simulink model "FA_18_MPC_Controller_2016b"  (R2016b)
settings: Solver=ode45  StartTime=0.0  StopTime=200  RelTol=1e-3
PreLoadFcn:
  | F18_Linear
values from neighbouring files (symbols this model uses):
  C1 = [0 -1 0 1]    [F18_Linear.m]
  d2r = pi/180    (= 0.0174532925199)    [F18_Linear.m]    (also in FA_18_Trim.m; FA_18_sfun.m; Sim.m)
  F1 = [-67.81 11973 -133.3 -11801]    [F18_Linear.m]
  F2 = 1414.2    [F18_Linear.m]
  Trimx_N = [365.74;15*d2r;0;15*d2r]    [F18_Linear.m]
undefined symbols (not defined in the file or in its folder): Earth, WGS84
libraries: simulink_extras x2, aerolibfltsims x1, mpclib x1, aerolibtransform2 x1, aerolibconvert2 x1
settings Model: Creator=User  LastModifiedBy=Amruth Nanjangud

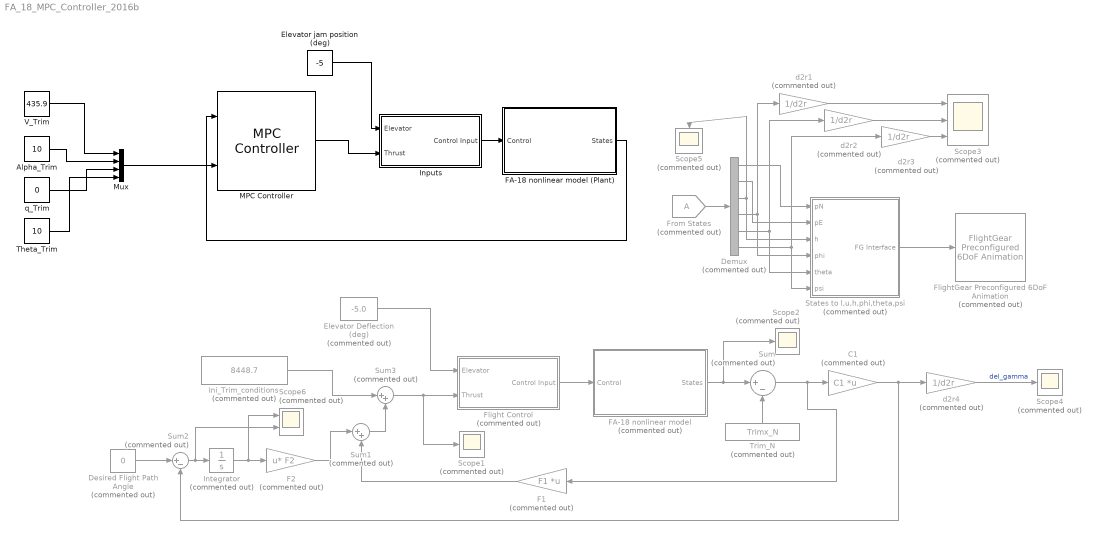
== system FA_18_MPC_Controller_2016b ==
  Alpha_Trim : Constant  Value=10
  C1 : Gain  Commented=on  Gain=C1  Multiplication=Matrix(K*u)
  Demux : Demux  Commented=on  Outputs=6
  Desired Flight Path Angle : Constant  Commented=on  Value=0
  Elevator Deflection (deg) : Constant  Commented=on  Value=-5.0
  Elevator jam position (deg) : Constant  Value=-5
  F1 : Gain  Commented=on  Gain=F1  Multiplication=Matrix(K*u)
  F2 : Gain  Commented=on  Gain=F2  Multiplication=Matrix(u*K)
  FA-18 nonlinear model : Subsystem  Commented=on
  FA-18 nonlinear model (Plant) : Subsystem
  Flight Control : Subsystem  Commented=on
  FlightGear Preconfigured 6DoF Animation : aerolibfltsims/FlightGear Preconfigured 6DoF Animation  Commented=on  xFlightGearVersion=v2016.1  DestinationIpAddress=127.0.0.1  DestinationPort=5502  SampleTime=1/30
  From States : From  Commented=on  TagVisibility=global
  Ini_Trim_conditions : Constant  Commented=on  Value=8448.7
  "Inputs " : Subsystem
  Integrator : Integrator  Commented=on
  MPC Controller : mpclib/MPC Controller  SCDEnableBlockLinearizationSpecification=on  mpcobj=mpc1  is_multiple=0  enable_value=0  return_u0=off  ref_from_ws=off  ref_signal_name=[]  ref_preview=off  md_from_ws=off  md_signal_name=[]  md_preview=off  from_project=off  project_file=MPCtask.mat  md_inport=off  mv_inport=off  cost_outport=off  return_sequence=off  return_qpstatus=off  return_state=off  state_inport=off  lims_inport=off  ywt_inport=off  is_designfromscratch=0  uwt_inport=off  duwt_inport=off  rhoeps_inport=off  uref_inport=off  n_ts=0.1  n_mv=1  n_md=0  n_ud=0  n_mo=4  n_uo=0  BlockDataType=double  SampleTimeInherited=off  switch_inport=off
  Mux : Mux
  Scope{1..2,4..5} (4 alike) : Scope  Commented=on
  Scope3 : Scope  Commented=on  NumInputPorts=3
  Scope6 : Scope  Commented=on  NumInputPorts=2
  States to l,u,h,phi,theta,psi : Subsystem  Commented=on
  Sum : Sum  Commented=on  Inputs=|+-
  Sum1 : Sum  Commented=on  Inputs=|++
  Sum2 : Sum  Commented=on  Inputs=|+-
  Sum3 : Sum  Commented=on  Inputs=|++
  Theta_Trim : Constant  Value=10
  Trim_N : Constant  Commented=on  Value=Trimx_N
  V_Trim : Constant  Value=435.9
  d2r{1..4} (4 alike) : Gain  Commented=on  Gain=1/d2r
  q_Trim : Constant  Value=0
  wires:
  Flight Control/1(Control Input) -> FA-18 nonlinear model/1(Control)
  Elevator Deflection (deg)/1 -> Flight Control/1(Elevator)
  FA-18 nonlinear model/1(States) -> Scope2/1, Sum/1
  Trim_N/1 -> Sum/2
  d2r4/1 -> Scope4/1  "del_gamma"
  Sum2/1 -> Scope6/2, Integrator/1
  Integrator/1 -> Scope6/1, F2/1
  Desired Flight Path Angle/1 -> Sum2/1
  C1/1 -> d2r4/1, Sum2/2
  F2/1 -> Sum1/1
  Sum1/1 -> Sum3/2
  F1/1 -> Sum1/2
  Sum3/1 -> Scope1/1, Flight Control/2(Thrust)
  Ini_Trim_conditions/1 -> Sum3/1
  Sum/1 -> F1/1, C1/1
  States to l,u,h,phi,theta,psi/1(FG Interface) -> FlightGear Preconfigured 6DoF Animation/1
  From States/1 -> Demux/1
  Demux/1 -> States to l,u,h,phi,theta,psi/1(pN)
  Demux/2 -> States to l,u,h,phi,theta,psi/2(pE)
  Demux/5 -> States to l,u,h,phi,theta,psi/5(theta), d2r2/1
  Demux/6 -> d2r3/1, States to l,u,h,phi,theta,psi/6(psi)
  Demux/4 -> d2r1/1, States to l,u,h,phi,theta,psi/4(phi)
  d2r1/1 -> Scope3/1
  d2r2/1 -> Scope3/2
  d2r3/1 -> Scope3/3
  Demux/3 -> Scope5/1, States to l,u,h,phi,theta,psi/3(h)
  "Inputs "/1(Control Input) -> FA-18 nonlinear model (Plant)/1(Control)
  MPC Controller/1 -> "Inputs "/2(Thrust)
  Elevator jam position (deg)/1 -> "Inputs "/1(Elevator)
  FA-18 nonlinear model (Plant)/1(States) -> MPC Controller/1
  Mux/1 -> MPC Controller/2
  V_Trim/1 -> Mux/1
  Alpha_Trim/1 -> Mux/2
  q_Trim/1 -> Mux/3
  Theta_Trim/1 -> Mux/4

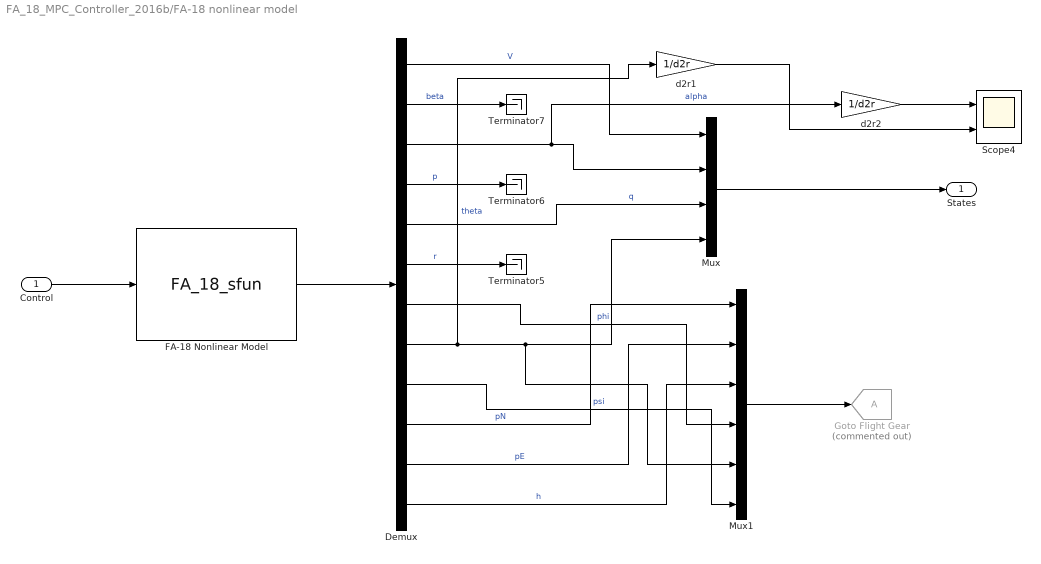
== system FA_18_MPC_Controller_2016b/FA-18 nonlinear model ==
  Control : Inport
  Demux : Demux  Outputs=12
  FA-18 Nonlinear Model : S-Function  FunctionName=FA_18_sfun  SFunctionDeploymentMode=off  EnableBusSupport=off
  Goto Flight Gear : Goto  Commented=on  TagVisibility=global
  Mux : Mux
  Mux1 : Mux  Inputs=6
  Scope4 : Scope  NumInputPorts=2
  Terminator5 : Terminator
  Terminator6 : Terminator
  Terminator7 : Terminator
  d2r1 : Gain  Gain=1/d2r
  d2r2 : Gain  Gain=1/d2r
  States : Outport
  wires:
  Control/1 -> FA-18 Nonlinear Model/1
  Demux/1 -> Mux/1  "V"
  FA-18 Nonlinear Model/1 -> Demux/1
  Demux/3 -> d2r2/1, Mux/2  "alpha"
  Demux/8 -> Mux1/5, Mux/4, d2r1/1  "theta"
  Demux/12 -> Mux1/3  "h"
  Demux/9 -> Mux1/6  "psi"
  Demux/11 -> Mux1/2  "pE"
  Demux/2 -> Terminator7/1  "beta"
  Demux/10 -> Mux1/1  "pN"
  Demux/6 -> Terminator5/1  "r"
  Demux/5 -> Mux/3  "q"
  Mux/1 -> States/1
  Demux/4 -> Terminator6/1  "p"
  Mux1/1 -> Goto Flight Gear/1
  Demux/7 -> Mux1/4  "phi"
  d2r1/1 -> Scope4/2
  d2r2/1 -> Scope4/1

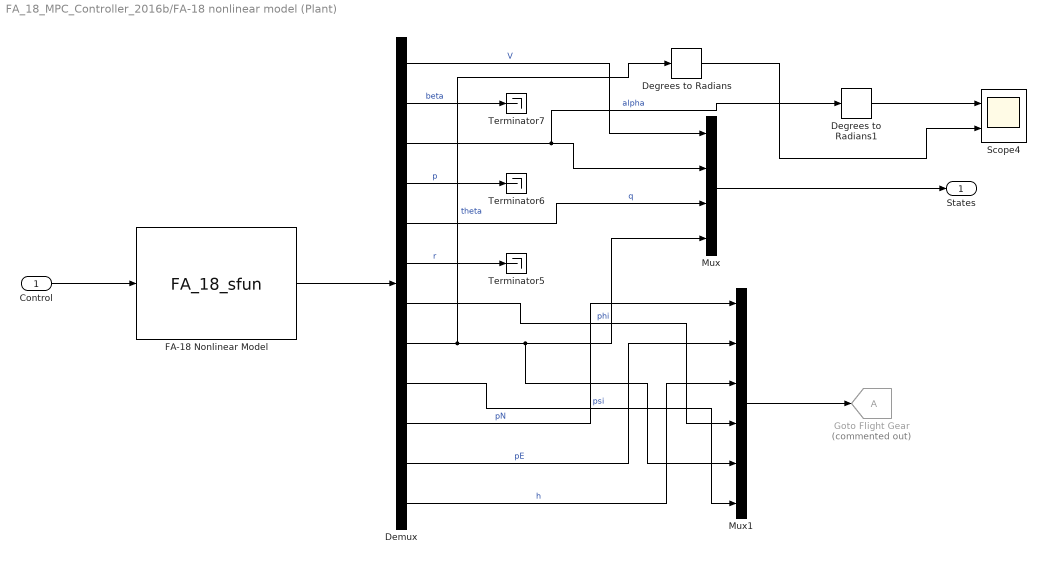
== system FA_18_MPC_Controller_2016b/FA-18 nonlinear model (Plant) ==
  Control : Inport
  Degrees to Radians : simulink_extras/Transformations/Degrees to Radians
  Degrees to Radians1 : simulink_extras/Transformations/Degrees to Radians
  Demux : Demux  Outputs=12
  FA-18 Nonlinear Model : S-Function  FunctionName=FA_18_sfun  SFunctionDeploymentMode=off  EnableBusSupport=off
  Goto Flight Gear : Goto  Commented=on  TagVisibility=global
  Mux : Mux
  Mux1 : Mux  Inputs=6
  Scope4 : Scope  NumInputPorts=2
  Terminator5 : Terminator
  Terminator6 : Terminator
  Terminator7 : Terminator
  States : Outport
  wires:
  Degrees to Radians1/1 -> Scope4/1
  Degrees to Radians/1 -> Scope4/2
  Demux/7 -> Mux1/4  "phi"
  Mux1/1 -> Goto Flight Gear/1
  Demux/4 -> Terminator6/1  "p"
  Mux/1 -> States/1
  Demux/5 -> Mux/3  "q"
  Demux/6 -> Terminator5/1  "r"
  Demux/10 -> Mux1/1  "pN"
  Demux/2 -> Terminator7/1  "beta"
  Demux/11 -> Mux1/2  "pE"
  Demux/9 -> Mux1/6  "psi"
  Demux/12 -> Mux1/3  "h"
  Demux/8 -> Degrees to Radians/1, Mux/4, Mux1/5  "theta"
  Demux/3 -> Degrees to Radians1/1, Mux/2  "alpha"
  FA-18 Nonlinear Model/1 -> Demux/1
  Demux/1 -> Mux/1  "V"
  Control/1 -> FA-18 Nonlinear Model/1

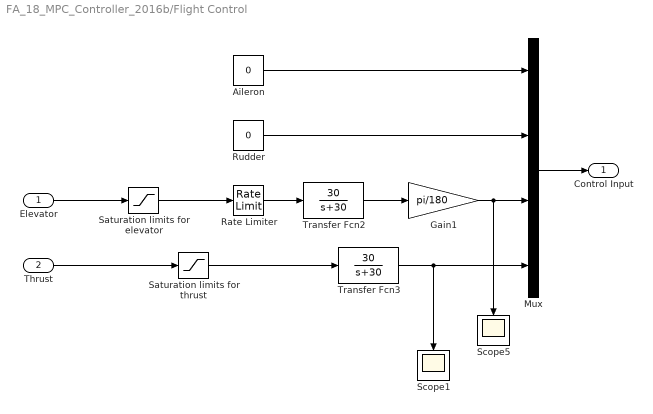
== system FA_18_MPC_Controller_2016b/Flight Control ==
  Elevator : Inport
  Thrust : Inport  Port=2
  Aileron : Constant  Value=0
  Gain1 : Gain  Gain=pi/180
  Mux : Mux
  Rate Limiter : RateLimiter  RisingSlewLimit=40  FallingSlewLimit=-40  SampleTimeMode=inherited
  Rudder : Constant  Value=0
  Saturation limits for elevator : Saturate  UpperLimit=10.5  LowerLimit=-24
  Saturation limits for thrust : Saturate  UpperLimit=20000  LowerLimit=0
  Scope1 : Scope
  Scope5 : Scope
  Transfer Fcn2 : TransferFcn  Numerator=[30]  Denominator=[1 30]
  Transfer Fcn3 : TransferFcn  Numerator=[30]  Denominator=[1 30]
  Control Input : Outport
  wires:
  Mux/1 -> Control Input/1
  Aileron/1 -> Mux/1
  Thrust/1 -> Saturation limits for thrust/1
  Transfer Fcn3/1 -> Scope1/1, Mux/4
  Rudder/1 -> Mux/2
  Saturation limits for thrust/1 -> Transfer Fcn3/1
  Saturation limits for elevator/1 -> Rate Limiter/1
  Rate Limiter/1 -> Transfer Fcn2/1
  Elevator/1 -> Saturation limits for elevator/1
  Gain1/1 -> Mux/3, Scope5/1
  Transfer Fcn2/1 -> Gain1/1

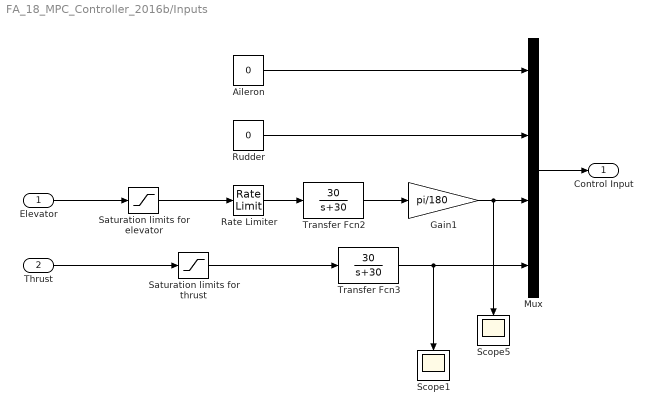
== system FA_18_MPC_Controller_2016b/Inputs  ==
  Elevator : Inport
  Thrust : Inport  Port=2
  Aileron : Constant  Value=0
  Gain1 : Gain  Gain=pi/180
  Mux : Mux
  Rate Limiter : RateLimiter  RisingSlewLimit=40  FallingSlewLimit=-40  SampleTimeMode=inherited
  Rudder : Constant  Value=0
  Saturation limits for elevator : Saturate  UpperLimit=10.5  LowerLimit=-24
  Saturation limits for thrust : Saturate  UpperLimit=20000  LowerLimit=0
  Scope1 : Scope
  Scope5 : Scope
  Transfer Fcn2 : TransferFcn  Numerator=[30]  Denominator=[1 30]
  Transfer Fcn3 : TransferFcn  Numerator=[30]  Denominator=[1 30]
  Control Input : Outport
  wires:
  Transfer Fcn2/1 -> Gain1/1
  Gain1/1 -> Scope5/1, Mux/3
  Elevator/1 -> Saturation limits for elevator/1
  Rate Limiter/1 -> Transfer Fcn2/1
  Saturation limits for elevator/1 -> Rate Limiter/1
  Saturation limits for thrust/1 -> Transfer Fcn3/1
  Rudder/1 -> Mux/2
  Transfer Fcn3/1 -> Mux/4, Scope1/1
  Thrust/1 -> Saturation limits for thrust/1
  Aileron/1 -> Mux/1
  Mux/1 -> Control Input/1

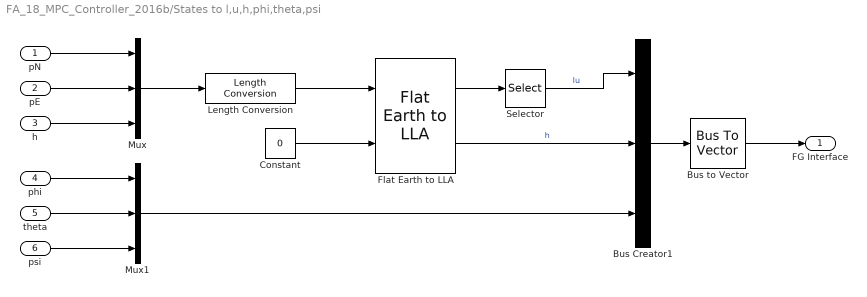
== system FA_18_MPC_Controller_2016b/States to l,u,h,phi,theta,psi ==
  pN : Inport
  pE : Inport  Port=2
  h : Inport  Port=3
  phi : Inport  Port=4
  theta : Inport  Port=5
  psi : Inport  Port=6
  Bus Creator1 : BusCreator  Inputs=3
  Bus to Vector : BusToVector
  Constant : Constant  Value=0
  Flat Earth to LLA : aerolibtransform2/Flat Earth to LLA  units=Metric (MKS)  ptype=Earth (WGS84)  F=1/298.257223563  R=6378137  LL0=[50.1018 14.2632]  psi=0
  Length Conversion : aerolibconvert2/Length Conversion  IU=ft  OU=m
  Mux : Mux  Inputs=3
  Mux1 : Mux  Inputs=3
  Selector : Selector  IndexMode=Zero-based  InputPortWidth=2  IndexOptions=Index vector (dialog)  Indices=[1 0]  OutputSizes=1
  FG Interface : Outport
  wires:
  Constant/1 -> Flat Earth to LLA/2
  Length Conversion/1 -> Flat Earth to LLA/1
  Bus to Vector/1 -> FG Interface/1
  Bus Creator1/1 -> Bus to Vector/1
  Flat Earth to LLA/1 -> Selector/1
  Selector/1 -> Bus Creator1/1  "lu"
  Flat Earth to LLA/2 -> Bus Creator1/2  "h"
  pN/1 -> Mux/1
  pE/1 -> Mux/2
  h/1 -> Mux/3
  Mux/1 -> Length Conversion/1
  theta/1 -> Mux1/2
  phi/1 -> Mux1/1
  psi/1 -> Mux1/3
  Mux1/1 -> Bus Creator1/3
